simulink model "UAV_modelo_naolinear_1"  (R2017a)
settings: Solver=ode23s  StartTime=0.0  StopTime=T_sim  RelTol=1e-3  EnableMultiTasking=on
InitFcn:
  | main_modelo_nao_linear_v1
values from neighbouring files (symbols this model uses):
  dphi0 = 0    [main_model1.m]    (also in main_modelo_nao_linear_v1.m)
  dpsi0 = 0    [main_model1.m]    (also in main_modelo_nao_linear_v1.m)
  dtheta0 = 0    [main_model1.m]    (also in main_modelo_nao_linear_v1.m)
  g = 9.8    [main_model1.m]    (also in main_model2.m; main_modelo_linear_v1.m; main_modelo_linear_v2.m; main_modelo_nao_linear_v1.m)
  incluir_din_motor = -1    [main_model1.m]    (also in main_model2.m; main_modelo_nao_linear_v1.m = 1; main_modelo_nao_linear_v2.m; modelo_naolinear.m = 1)
  Ir = 1e-3    (= 0.001)    [main_model1.m]    (also in main_model2.m; main_modelo_linear_v1.m = 0.01; main_modelo_linear_v2.m = 0.01; main_modelo_nao_linear_v1.m)
  Ixx = 1e-2    (= 0.01)    [main_model1.m]    (also in main_model2.m; main_modelo_linear_v1.m; main_modelo_linear_v2.m; main_modelo_nao_linear_v1.m)
  Iyy = 1e-2    (= 0.01)    [main_model1.m]    (also in main_model2.m; main_modelo_linear_v1.m; main_modelo_linear_v2.m; main_modelo_nao_linear_v1.m)
  Izz = 1.8e-2    (= 0.018)    [main_model1.m]    (also in main_model2.m; main_modelo_linear_v1.m; main_modelo_linear_v2.m; main_modelo_nao_linear_v1.m)
  Kd_rot = 0.01    [main_model1.m]    (also in main_model2.m; main_modelo_linear_v1.m = 0; main_modelo_linear_v2.m = 0; main_modelo_nao_linear_v1.m)
  Kd_trans = 0.002    [main_model1.m]    (also in main_model2.m = -0.13723; main_modelo_linear_v1.m = 0; main_modelo_linear_v2.m = 0; main_modelo_nao_linear_v1.m)
  Ki_rot = 1.0    (= 1)    [main_model1.m]    (also in main_model2.m; main_modelo_linear_v1.m = 0.5; main_modelo_linear_v2.m = 0.5; main_modelo_nao_linear_v1.m)
  Ki_trans = 0.06    [main_model1.m]    (also in main_model2.m = 0.41774; main_modelo_linear_v1.m = 0; main_modelo_linear_v2.m = 1; main_modelo_nao_linear_v1.m)
  Kp = 0.9182    [main_model1.m]    (also in main_model2.m; main_modelo_nao_linear_v1.m; main_modelo_nao_linear_v2.m; modelo_naolinear.m)
  Kp_rot = 10    [main_model1.m]    (also in main_model2.m; main_modelo_linear_v1.m = 1; main_modelo_linear_v2.m = 1; main_modelo_nao_linear_v1.m)
  Kp_trans = 0.4    [main_model1.m]    (also in main_model2.m = 2.0968; main_modelo_linear_v1.m = 1; main_modelo_linear_v2.m = 2; main_modelo_nao_linear_v1.m)
  m = 1.0428    [main_model1.m]    (also in main_model2.m; main_modelo_linear_v1.m = 1; main_modelo_linear_v2.m = 1; main_modelo_nao_linear_v1.m)
  phi0 = 0    [main_model1.m]    (also in main_model2.m; main_modelo_linear_v1.m; main_modelo_linear_v2.m; main_modelo_nao_linear_v1.m)
  psi0 = 0    [main_model1.m]    (also in main_model2.m; main_modelo_linear_v1.m; main_modelo_linear_v2.m; main_modelo_nao_linear_v1.m)
  T = [kf,kf,kf,kf ... (first row only)    [main_model1.m]    (also in main_model2.m; main_modelo_nao_linear_v1.m; main_modelo_nao_linear_v2.m; modelo_naolinear.m)
  T_inv = T^(-1)    [main_model1.m]    (also in main_model2.m; main_modelo_nao_linear_v1.m; main_modelo_nao_linear_v2.m; modelo_naolinear.m)
  tau_a = 0.0569    [main_model1.m]    (also in main_model2.m; main_modelo_nao_linear_v1.m; main_modelo_nao_linear_v2.m; modelo_naolinear.m)
  tau_s = 0.0452    [main_model1.m]    (also in main_model2.m; main_modelo_nao_linear_v1.m; main_modelo_nao_linear_v2.m; modelo_naolinear.m)
  theta0 = 0    [main_model1.m]    (also in main_model2.m; main_modelo_linear_v1.m; main_modelo_linear_v2.m; main_modelo_nao_linear_v1.m)
  vx0 = 0    [main_model1.m]    (also in main_model2.m; main_modelo_nao_linear_v1.m; main_modelo_nao_linear_v2.m; modelo_naolinear.m)
  vxd = 0    [main_model1.m]    (also in main_model2.m; main_modelo_linear_v1.m; main_modelo_linear_v2.m; main_modelo_nao_linear_v1.m)
  vy0 = 0    [main_model1.m]    (also in main_model2.m; main_modelo_nao_linear_v1.m; main_modelo_nao_linear_v2.m; modelo_naolinear.m)
  vyd = 0    [main_model1.m]    (also in main_model2.m; main_modelo_linear_v1.m; main_modelo_linear_v2.m; main_modelo_nao_linear_v1.m)
  vz0 = 0    [main_model1.m]    (also in main_model2.m; main_modelo_nao_linear_v1.m; main_modelo_nao_linear_v2.m; modelo_naolinear.m)
  x0 = 0    [main_model1.m]    (also in main_model2.m; main_modelo_linear_v1.m; main_modelo_linear_v2.m; main_modelo_nao_linear_v1.m)
  y0 = 0    [main_model1.m]    (also in main_model2.m; main_modelo_linear_v1.m; main_modelo_linear_v2.m; main_modelo_nao_linear_v1.m)
  z0 = 1    [main_model1.m]    (also in main_model2.m; main_modelo_linear_v1.m; main_modelo_linear_v2.m; main_modelo_nao_linear_v1.m)
undefined symbols (not defined in the file or in its folder): sigbuilder_block
libraries: simulink x6, vrlib x2, aerolibutil x2, sharedutil x1
settings Model: Creator=dferr  LastModifiedBy=diego
settings DataIOCC: LimitDataPoints=on  SaveFormat=Array
settings OptimizationCC: LifeSpan=inf
settings DebuggingCC: SFUnexpectedBacktrackingDiag=warning  SFNoUnconditionalDefaultTransitionDiag=warning  SFExecutionAtInitializationDiag=none
settings HardwareCC: ProdBitPerPointer=32  ProdBitPerSizeT=32  ProdBitPerPtrDiffT=32  ProdLargestAtomicFloat=None  ProdIntDivRoundTo=Undefined  ProdEndianess=Unspecified  ProdWordSize=32  ProdHWDeviceType=32-bit Generic
settings ModelReferenceCC: PropagateSignalLabelsOutOfModel=off
settings GRTTargetCC: TargetLangStandard=C89/C90 (ANSI)  GeneratePreprocessorConditionals=Disable all
settings ConfigComp: CovMetricSettings=dw  CovHtmlReporting=on  CovSaveCumulativeToWorkspaceVar=on  CovSaveSingleToWorkspaceVar=on  CovExternalEMLEnable=off  CovSFcnEnable=off

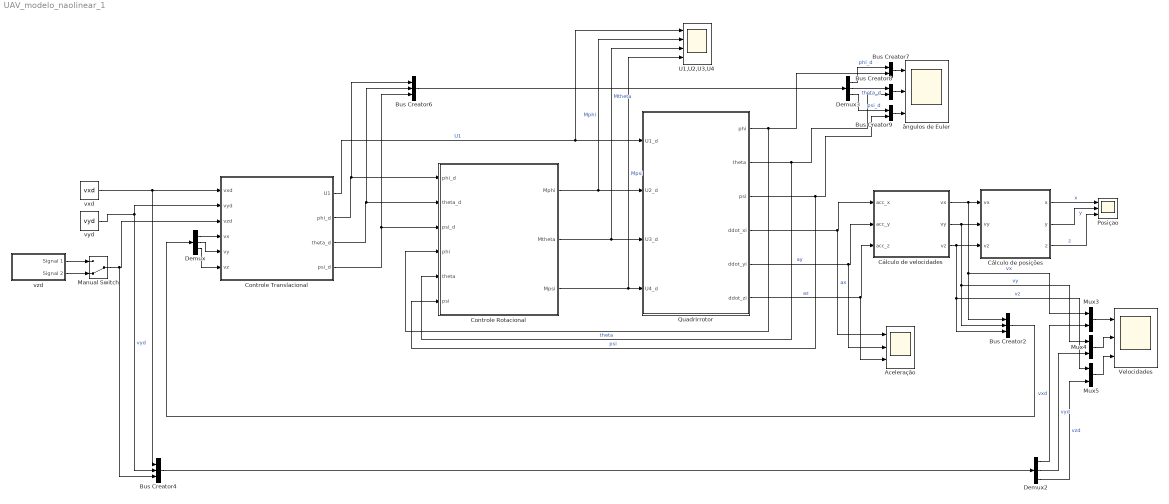
== system UAV_modelo_naolinear_1 ==
  Aceleração : Scope  NumInputPorts=3
  Bus Creator2 : BusCreator  Inputs=3
  Bus Creator4 : BusCreator  Inputs=3
  Bus Creator6 : BusCreator  Inputs=3
  Bus Creator7 : BusCreator  Inputs=2
  Bus Creator8 : BusCreator  Inputs=2
  Bus Creator9 : BusCreator  Inputs=2
  Controle Rotacional : Subsystem
      mask Display:
      | disp('Controle Rotacional')
      | port_label('input',1,'phi_d')
      | port_label('input',2,'theta_d')
      | port_label('input',3,'psi_d')
      | port_label('input',4,'phi')
      | port_label('input',5,'theta')
      | port_label('input',6,'psi')
      | port_label('output',1,'Mphi')
      | port_label('output',2,'Mtheta')
      | port_label('output',3,'Mpsi')
  Controle Translacional : Subsystem
      mask Display:
      | disp('Controle Translacional')
      | port_label('input',1,'vxd')
      | port_label('input',2,'vyd')
      | port_label('input',3,'vzd')
      | port_label('input',4,'vx')
      | port_label('input',5,'vy')
      | port_label('input',6,'vz')
      | port_label('output',1,'U1')
      | port_label('output',2,'phi_d')
      | port_label('output',3,'theta_d')
      | port_label('output',4,'psi_d')
  Cálculo de posições : Subsystem
      mask Display:
      | disp('Vel -> Pos')
      | port_label('input',1,'vel_x')
      | port_label('input',2,'vel_y')
      | port_label('input',3,'vel_ z')
      | port_label('output',1,'x')
      | port_label('output',2,'y')
      | port_label('output',3,'z')
  Cálculo de velocidades : Subsystem
      mask Display:
      | disp('Acc -> Vel')
      | port_label('input',1,'acc_x')
      | port_label('input',2,'acc_y')
      | port_label('input',3,'acc_z')
      | port_label('output',1,'vel_x')
      | port_label('output',2,'vel_y')
      | port_label('output',3,'vel_z')
  Demux : Demux  Outputs=3
  Demux2 : Demux  Outputs=3
  Demux3 : Demux  Outputs=3
  Manual Switch : ManualSwitch  CurrentSetting=0
  Mux3 : Mux  Inputs=2
  Mux4 : Mux  Inputs=2
  Mux5 : Mux  Inputs=2
  Posiçao : Scope  NumInputPorts=3
  Quadrirrotor : Subsystem
      mask Display:
      | disp('Quadrirrotor')
      | port_label('input',1,'U1')
      | port_label('input',2,'U2')
      | port_label('input',3,'U3')
      | port_label('input',4,'U4')
      | port_label('output',1,'phi')
      | port_label('output',2,'theta')
      | port_label('output',3,'psi')
      | port_label('output',4,'ddot_xi')
      | port_label('output',5,'ddot_yi')
      | port_label('output',6,'ddot_zi')
  U1,U2,U3,U4 : Scope  NumInputPorts=4
  Velocidades : Scope  NumInputPorts=3
  vxd : Constant  Value=vxd
  vyd : Constant  Value=vyd
  vzd : Subsystem  Tag=STV Subsys  LoadFcn=sigbuilder_block('load');  StartFcn=sigbuilder_block('start');  StopFcn=sigbuilder_block('stop');  ClipboardFcn=sigbuilder_block('clipboard');  mask(Sigbuilder block){tuvar=[0:10]}
      mask help: Simulink:masks:SigbuilderBlock_MD
      mask init:
      | if ~strcmp(get_param(bdroot(gcbh),'SimulationStatus'),'stopped') tuvar = sigbuilder_block('maskInit'); end
      settings: CopyFcn=sigbuilder_block('copy');  DeleteFcn=sigbuilder_block('delete');  ModelCloseFcn=sigbuilder_block('modelClose');  PreSaveFcn=sigbuilder_block('preSave');  PauseFcn=sigbuilder_block('pause');  ContinueFcn=sigbuilder_block('continue');  NameChangeFcn=sigbuilder_block('namechange');  OpenFcn=sigbuilder_block('open',[437.76 199.44 550.08 399.6 ]);  CloseFcn=sigbuilder_block('close');
      mask Display: plot(0, 0, 100, 100,[2, 2, 32, 32, 2], [68, 8, 8, 68, 68],[32, 2], [38, 38], [32, 19, 2],[53, 60, 44], [32, 17, 17, 2],[16, 16, 31, 31]);txt = getActiveGroup(gcbh);text(2, 100, txt,'verticalAlignment', 'top');
  ângulos de Euler : Scope  NumInputPorts=3
  wires:
  Cálculo de velocidades/1(vx) -> Mux3/1, Bus Creator2/1, Cálculo de posições/1(vx)  "vx"
  Cálculo de velocidades/2(vy) -> Mux4/1, Bus Creator2/2, Cálculo de posições/2(vy)  "vy"
  Cálculo de velocidades/3(vz) -> Mux5/1, Bus Creator2/3, Cálculo de posições/3(vz)  "vz"
  Bus Creator2/1 -> Demux/1
  vyd/1 -> Controle Translacional/2(vyd), Bus Creator4/2  "vyd"
  Mux3/1 -> Velocidades/1
  Mux4/1 -> Velocidades/2
  Mux5/1 -> Velocidades/3
  Bus Creator4/1 -> Demux2/1
  Demux2/1 -> Mux3/2  "vxd"
  Demux2/2 -> Mux4/2  "vyd"
  Demux2/3 -> Mux5/2  "vzd"
  Controle Rotacional/1(Mphi) -> U1,U2,U3,U4/2, Quadrirrotor/2(U2_d)  "Mphi"
  Controle Rotacional/2(Mtheta) -> U1,U2,U3,U4/3, Quadrirrotor/3(U3_d)  "Mtheta"
  Controle Rotacional/3(Mpsi) -> U1,U2,U3,U4/4, Quadrirrotor/4(U4_d)  "Mpsi"
  Quadrirrotor/1(phi) -> Controle Rotacional/4(phi), Bus Creator7/2
  Quadrirrotor/2(theta) -> Controle Rotacional/5(theta), Bus Creator8/2  "theta"
  Quadrirrotor/3(psi) -> Controle Rotacional/6(psi), Bus Creator9/2  "psi"
  Quadrirrotor/4(ddot_xi) -> Aceleração/1, Cálculo de velocidades/1(acc_x)  "ax"
  Quadrirrotor/5(ddot_yi) -> Aceleração/2, Cálculo de velocidades/2(acc_y)  "ay"
  Quadrirrotor/6(ddot_zi) -> Aceleração/3, Cálculo de velocidades/3(acc_z)  "az"
  Demux/1 -> Controle Translacional/4(vx)
  Demux/2 -> Controle Translacional/5(vy)
  Demux/3 -> Controle Translacional/6(vz)
  Controle Translacional/1(U1) -> U1,U2,U3,U4/1, Quadrirrotor/1(U1_d)  "U1"
  Controle Translacional/2(phi_d) -> Controle Rotacional/1(phi_d), Bus Creator6/1
  Controle Translacional/3(theta_d) -> Controle Rotacional/2(theta_d), Bus Creator6/2
  Controle Translacional/4(psi_d) -> Bus Creator6/3, Controle Rotacional/3(psi_d)
  Bus Creator6/1 -> Demux3/1
  Bus Creator7/1 -> ângulos de Euler/1
  Bus Creator8/1 -> ângulos de Euler/2
  Bus Creator9/1 -> ângulos de Euler/3
  Demux3/1 -> Bus Creator7/1  "phi_d"
  Demux3/2 -> Bus Creator8/1  "theta_d"
  Demux3/3 -> Bus Creator9/1  "psi_d"
  vxd/1 -> Bus Creator4/1, Controle Translacional/1(vxd)
  Cálculo de posições/1(x) -> Posiçao/1  "x"
  Cálculo de posições/2(y) -> Posiçao/2  "y"
  Cálculo de posições/3(z) -> Posiçao/3  "z"
  Manual Switch/1 -> Bus Creator4/3, Controle Translacional/3(vzd)
  vzd/1(Signal 1) -> Manual Switch/1
  vzd/2(Signal 2) -> Manual Switch/2

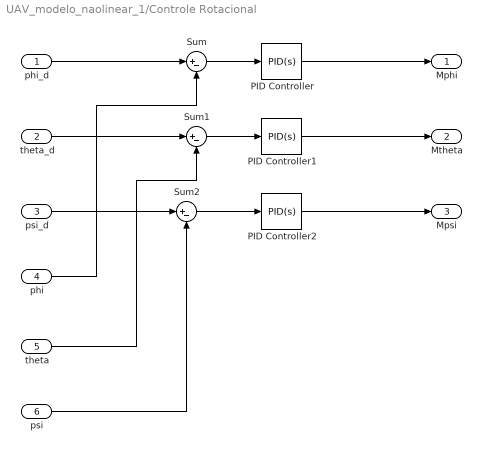
== system UAV_modelo_naolinear_1/Controle Rotacional ==
  phi_d : Inport
  theta_d : Inport  Port=2
  psi_d : Inport  Port=3
  phi : Inport  Port=4
  theta : Inport  Port=5
  psi : Inport  Port=6
  PID Controller : simulink/Continuous/PID Controller  Controller=PID  TimeDomain=Continuous-time  SampleTime=-1  IntegratorMethod=Forward Euler  FilterMethod=Forward Euler  Form=Parallel  UseFilter=on  ControllerParametersSource=internal  P=Kp_rot  I=Ki_rot  D=Kd_rot  N=100  InitialConditionSource=internal  InitialConditionForIntegrator=0  InitialConditionForFilter=0  ExternalReset=none  LimitOutput=off  UpperSaturationLimit=inf  LowerSaturationLimit=-inf  LinearizeAsGain=on  AntiWindupMode=none  Kb=1  TrackingMode=off  Kt=1  PParamMin=[]  PParamMax=[]  IParamMin=[]  IParamMax=[]  DParamMin=[]  DParamMax=[]  NParamMin=[]  NParamMax=[]  KbParamMin=[]  KbParamMax=[]  KtParamMin=[]  KtParamMax=[]  POutMin=[]  POutMax=[]  IOutMin=[]  IOutMax=[]  DOutMin=[]  DOutMax=[]  NOutMin=[]  NOutMax=[]  KbOutMin=[]  KbOutMax=[]  KtOutMin=[]  KtOutMax=[]  IntegratorOutMin=[]  IntegratorOutMax=[]  FilterOutMin=[]  FilterOutMax=[]  SumOutMin=[]  SumOutMax=[]  SumI1OutMin=[]  SumI1OutMax=[]  SumI2OutMin=[]  SumI2OutMax=[]  SumI3OutMin=[]  SumI3OutMax=[]  SumDOutMin=[]  SumDOutMax=[]  SaturationOutMin=[]  SaturationOutMax=[]  IntegratorContinuousStateAttributes=''  IntegratorStateMustResolveToSignalObject=off  IntegratorRTWStateStorageClass=Auto  FilterContinuousStateAttributes=''  FilterStateMustResolveToSignalObject=off  FilterRTWStateStorageClass=Auto  DifferentiatorICPrevScaledInput=0  DifferentiatorOutMin=[]  DifferentiatorOutMax=[]  InitialConditionSetting=State (most efficient)
  PID Controller1 : simulink/Continuous/PID Controller  Controller=PID  TimeDomain=Continuous-time  SampleTime=-1  IntegratorMethod=Forward Euler  FilterMethod=Forward Euler  Form=Parallel  UseFilter=on  ControllerParametersSource=internal  P=Kp_rot  I=Ki_rot  D=Kd_rot  N=100  InitialConditionSource=internal  InitialConditionForIntegrator=0  InitialConditionForFilter=0  ExternalReset=none  LimitOutput=off  UpperSaturationLimit=inf  LowerSaturationLimit=-inf  LinearizeAsGain=on  AntiWindupMode=none  Kb=1  TrackingMode=off  Kt=1  PParamMin=[]  PParamMax=[]  IParamMin=[]  IParamMax=[]  DParamMin=[]  DParamMax=[]  NParamMin=[]  NParamMax=[]  KbParamMin=[]  KbParamMax=[]  KtParamMin=[]  KtParamMax=[]  POutMin=[]  POutMax=[]  IOutMin=[]  IOutMax=[]  DOutMin=[]  DOutMax=[]  NOutMin=[]  NOutMax=[]  KbOutMin=[]  KbOutMax=[]  KtOutMin=[]  KtOutMax=[]  IntegratorOutMin=[]  IntegratorOutMax=[]  FilterOutMin=[]  FilterOutMax=[]  SumOutMin=[]  SumOutMax=[]  SumI1OutMin=[]  SumI1OutMax=[]  SumI2OutMin=[]  SumI2OutMax=[]  SumI3OutMin=[]  SumI3OutMax=[]  SumDOutMin=[]  SumDOutMax=[]  SaturationOutMin=[]  SaturationOutMax=[]  IntegratorContinuousStateAttributes=''  IntegratorStateMustResolveToSignalObject=off  IntegratorRTWStateStorageClass=Auto  FilterContinuousStateAttributes=''  FilterStateMustResolveToSignalObject=off  FilterRTWStateStorageClass=Auto  DifferentiatorICPrevScaledInput=0  DifferentiatorOutMin=[]  DifferentiatorOutMax=[]  InitialConditionSetting=State (most efficient)
  PID Controller2 : simulink/Continuous/PID Controller  Controller=PID  TimeDomain=Continuous-time  SampleTime=-1  IntegratorMethod=Forward Euler  FilterMethod=Forward Euler  Form=Parallel  UseFilter=on  ControllerParametersSource=internal  P=Kp_rot  I=Ki_rot  D=Kd_rot  N=100  InitialConditionSource=internal  InitialConditionForIntegrator=0  InitialConditionForFilter=0  ExternalReset=none  LimitOutput=off  UpperSaturationLimit=inf  LowerSaturationLimit=-inf  LinearizeAsGain=on  AntiWindupMode=none  Kb=1  TrackingMode=off  Kt=1  PParamMin=[]  PParamMax=[]  IParamMin=[]  IParamMax=[]  DParamMin=[]  DParamMax=[]  NParamMin=[]  NParamMax=[]  KbParamMin=[]  KbParamMax=[]  KtParamMin=[]  KtParamMax=[]  POutMin=[]  POutMax=[]  IOutMin=[]  IOutMax=[]  DOutMin=[]  DOutMax=[]  NOutMin=[]  NOutMax=[]  KbOutMin=[]  KbOutMax=[]  KtOutMin=[]  KtOutMax=[]  IntegratorOutMin=[]  IntegratorOutMax=[]  FilterOutMin=[]  FilterOutMax=[]  SumOutMin=[]  SumOutMax=[]  SumI1OutMin=[]  SumI1OutMax=[]  SumI2OutMin=[]  SumI2OutMax=[]  SumI3OutMin=[]  SumI3OutMax=[]  SumDOutMin=[]  SumDOutMax=[]  SaturationOutMin=[]  SaturationOutMax=[]  IntegratorContinuousStateAttributes=''  IntegratorStateMustResolveToSignalObject=off  IntegratorRTWStateStorageClass=Auto  FilterContinuousStateAttributes=''  FilterStateMustResolveToSignalObject=off  FilterRTWStateStorageClass=Auto  DifferentiatorICPrevScaledInput=0  DifferentiatorOutMin=[]  DifferentiatorOutMax=[]  InitialConditionSetting=State (most efficient)
  Sum : Sum  Inputs=|+-
  Sum1 : Sum  Inputs=|+-
  Sum2 : Sum  Inputs=|+-
  Mphi : Outport
  Mtheta : Outport  Port=2
  Mpsi : Outport  Port=3
  wires:
  Sum/1 -> PID Controller/1
  phi_d/1 -> Sum/1
  Sum1/1 -> PID Controller1/1
  Sum2/1 -> PID Controller2/1
  theta_d/1 -> Sum1/1
  psi_d/1 -> Sum2/1
  phi/1 -> Sum/2
  theta/1 -> Sum1/2
  psi/1 -> Sum2/2
  PID Controller/1 -> Mphi/1
  PID Controller1/1 -> Mtheta/1
  PID Controller2/1 -> Mpsi/1

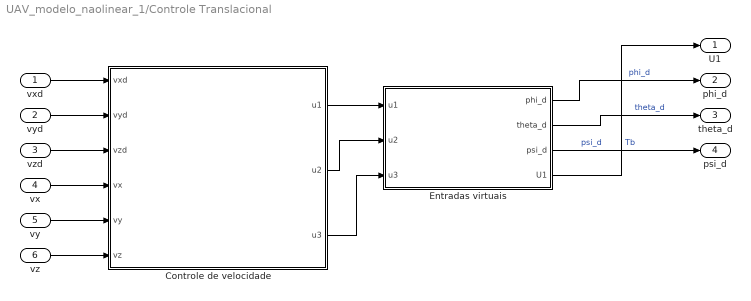
== system UAV_modelo_naolinear_1/Controle Translacional ==
  vxd : Inport
  vyd : Inport  Port=2
  vzd : Inport  Port=3
  vx : Inport  Port=4
  vy : Inport  Port=5
  vz : Inport  Port=6
  Controle de velocidade : Subsystem
      mask Display:
      | disp('Controle de Velocidade PID')
      | port_label('input',1,'vxd')
      | port_label('input',2,'vyd')
      | port_label('input',3,'vzd')
      | port_label('input',4,'vx')
      | port_label('input',5,'vy')
      | port_label('input',6,'vz')
      | 
      | port_label('output',1,'u1')
      | port_label('output',2,'u2')
      | port_label('output',3,'u3')
  Entradas virtuais : Subsystem
      mask Display:
      | disp('(u1,u2,u3)->(eta_d,U1)')
      | port_label('input',1,'u1')
      | port_label('input',2,'u2')
      | port_label('input',3,'u3')
      | port_label('output',1,'phi_d')
      | port_label('output',2,'theta_d')
      | port_label('output',3,'psi_d')
      | port_label('output',4,'U1')
  U1 : Outport
  phi_d : Outport  Port=2
  theta_d : Outport  Port=3
  psi_d : Outport  Port=4
  wires:
  Controle de velocidade/2(u2) -> Entradas virtuais/2(u2)
  Entradas virtuais/1(phi_d) -> phi_d/1  "phi_d"
  Entradas virtuais/2(theta_d) -> theta_d/1  "theta_d"
  Entradas virtuais/3(psi_d) -> psi_d/1  "psi_d"
  Controle de velocidade/1(u1) -> Entradas virtuais/1(u1)
  vz/1 -> Controle de velocidade/6(vz)
  vy/1 -> Controle de velocidade/5("vy ")
  Controle de velocidade/3(u3) -> Entradas virtuais/3(u3)
  vx/1 -> Controle de velocidade/4(vx)
  Entradas virtuais/4(U1) -> U1/1  "Tb"
  vyd/1 -> Controle de velocidade/2(vyd)
  vzd/1 -> Controle de velocidade/3(vzd)
  vxd/1 -> Controle de velocidade/1(vxd)

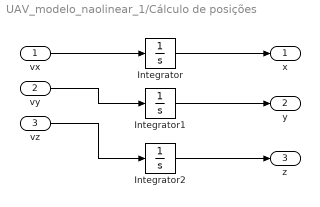
== system UAV_modelo_naolinear_1/Cálculo de posições ==
  vx : Inport
  vy : Inport  Port=2
  vz : Inport  Port=3
  Integrator : Integrator  InitialCondition=x0
  Integrator1 : Integrator  InitialCondition=y0
  Integrator2 : Integrator  InitialCondition=z0  LimitOutput=on  LowerSaturationLimit=0
  x : Outport
  y : Outport  Port=2
  z : Outport  Port=3
  wires:
  Integrator/1 -> x/1
  Integrator1/1 -> y/1
  vy/1 -> Integrator1/1
  vz/1 -> Integrator2/1
  vx/1 -> Integrator/1
  Integrator2/1 -> z/1

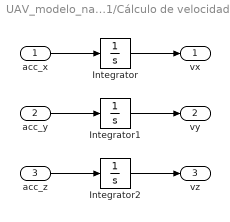
== system UAV_modelo_naolinear_1/Cálculo de velocidades ==
  acc_x : Inport
  acc_y : Inport  Port=2
  acc_z : Inport  Port=3
  Integrator : Integrator  InitialCondition=vx0  ZeroCross=off
  Integrator1 : Integrator  InitialCondition=vy0  ZeroCross=off
  Integrator2 : Integrator  InitialCondition=vz0  ZeroCross=off
  vx : Outport
  vy : Outport  Port=2
  vz : Outport  Port=3
  wires:
  Integrator2/1 -> vz/1
  acc_z/1 -> Integrator2/1
  Integrator/1 -> vx/1
  acc_x/1 -> Integrator/1
  acc_y/1 -> Integrator1/1
  Integrator1/1 -> vy/1

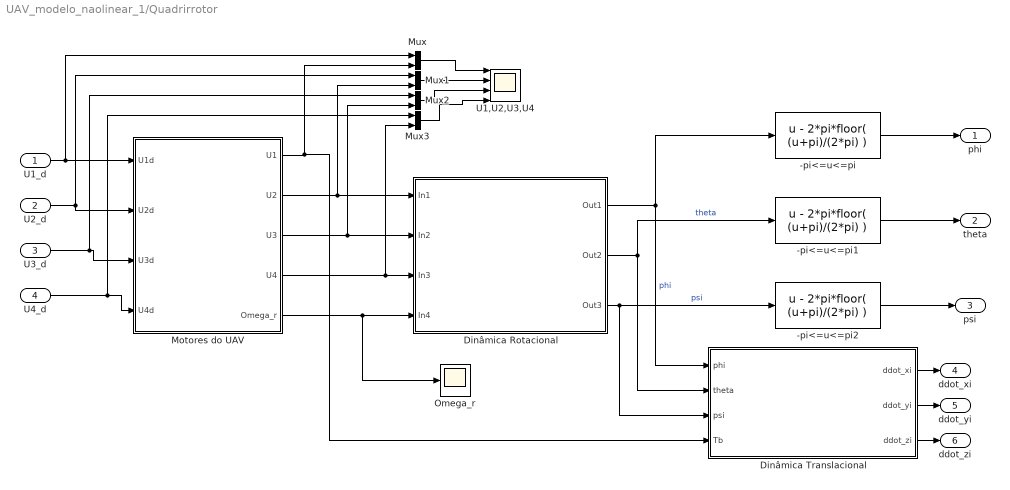
== system UAV_modelo_naolinear_1/Quadrirrotor ==
  U1_d : Inport
  U2_d : Inport  Port=2
  U3_d : Inport  Port=3
  U4_d : Inport  Port=4
  -pi<=u<=pi : Fcn  Expr=u - 2*pi*floor( (u+pi)/(2*pi) )
  -pi<=u<=pi1 : Fcn  Expr=u - 2*pi*floor( (u+pi)/(2*pi) )
  -pi<=u<=pi2 : Fcn  Expr=u - 2*pi*floor( (u+pi)/(2*pi) )
  Dinâmica Rotacional : Subsystem
      mask Display:
      | disp('Dinâmica Rotacional')
      | port_label('input',1,'Mphi')
      | port_label('input',2,'Mtheta')
      | port_label('input',3,'Mpsi')
      | port_label('input',4,'Omega_r')
      | port_label('output',1,'phi')
      | port_label('output',2,'theta')
      | port_label('output',3,'psi')
  Dinâmica Translacional : Subsystem
      mask Display:
      | disp ('Dinâmica Translacional')
      | port_label('input',1,'phi')
      | port_label('input',2,'theta')
      | port_label('input',3,'psi')
      | port_label('input',4,'Tb')
      | port_label('output',1,'ddot_xi')
      | port_label('output',2,'ddot_yi')
      | port_label('output',3,'ddot_zi')
  "Motores do UAV " : Subsystem
      mask Display:
      | disp('Dinâmica Motores')
      | port_label('input',1,'U1d')
      | port_label('input',2,'U2d')
      | port_label('input',3,'U3d')
      | port_label('input',4,'U4d')
      | port_label('output',1,'U1')
      | port_label('output',2,'U2')
      | port_label('output',3,'U3')
      | port_label('output',4,'U4')
      | port_label('output',5,'Omega_r')
  Mux{,1..3} (4 alike) : Mux  Inputs=2
  Omega_r : Scope
  U1,U2,U3,U4 : Scope  NumInputPorts=4
  phi : Outport
  theta : Outport  Port=2
  psi : Outport  Port=3
  ddot_xi : Outport  Port=4
  ddot_yi : Outport  Port=5
  ddot_zi : Outport  Port=6
  wires:
  Dinâmica Rotacional/3(Out3) -> Dinâmica Translacional/3(psi), -pi<=u<=pi2/1  "psi"
  Dinâmica Rotacional/2(Out2) -> Dinâmica Translacional/2(theta), -pi<=u<=pi1/1  "theta"
  Dinâmica Rotacional/1(Out1) -> Dinâmica Translacional/1(phi), -pi<=u<=pi/1  "phi"
  Dinâmica Translacional/1(ddot_xi) -> ddot_xi/1
  Dinâmica Translacional/2(ddot_yi) -> ddot_yi/1
  Dinâmica Translacional/3(ddot_zi) -> ddot_zi/1
  U2_d/1 -> "Motores do UAV "/2(U2d), Mux1/1
  U3_d/1 -> "Motores do UAV "/3(U3d), Mux2/1
  Mux/1 -> U1,U2,U3,U4/1
  Mux1/1 -> U1,U2,U3,U4/2
  Mux2/1 -> U1,U2,U3,U4/3
  Mux3/1 -> U1,U2,U3,U4/4
  "Motores do UAV "/3(U3) -> Dinâmica Rotacional/2(In2), Mux2/2
  "Motores do UAV "/4(U4) -> Mux3/2, Dinâmica Rotacional/3(In3)
  "Motores do UAV "/2(U2) -> Dinâmica Rotacional/1(In1), Mux1/2
  "Motores do UAV "/1(U1) -> Mux/2, Dinâmica Translacional/4(Tb)
  U1_d/1 -> "Motores do UAV "/1(U1d), Mux/1
  U4_d/1 -> "Motores do UAV "/4(U4d), Mux3/1
  "Motores do UAV "/5(Omega_r) -> Omega_r/1, Dinâmica Rotacional/4(In4)
  -pi<=u<=pi/1 -> phi/1
  -pi<=u<=pi1/1 -> theta/1
  -pi<=u<=pi2/1 -> psi/1

== system UAV_modelo_naolinear_1/vzd ==
  Demux : Demux  Tag=STV Demux  Outputs=2
  FromWs : FromWorkspace  Tag=STV FromWs  VariableName=tuvar  SampleTime=0
      SigBuilderData=|
      | common.afterFinalStr = 'Extrapolate'
      | common.sampleTime = 0
      | dataSet.timeRange = [0 20]
      | dataSet.name = 'Group 1'
      | sbobj.Groups.Name = 'Group 1'
      | sbobj.Groups.Signals(1).Name = 'Signal 1'
      | sbobj.Groups.Signals(1).XData = [0 2.05 4.75 8 18 20]
      | sbobj.Groups.Signals(1).YData = [-0.2 8.5 20 20 0 0]
      | sbobj.Groups.Signals(2).Name = 'Signal 2'
      | sbobj.Groups.Signals(2).XData = [0 5 5 20]
      | sbobj.Groups.Signals(2).YData = [0 0 1 1]
      | sbobj.Groups.TimeRange = [0 20]
  Signal 1 : Outport  Tag=STV Outport
  Signal 2 : Outport  Tag=STV Outport  Port=2
  wires:
  FromWs/1 -> Demux/1
  Demux/1 -> Signal 1/1
  Demux/2 -> Signal 2/1

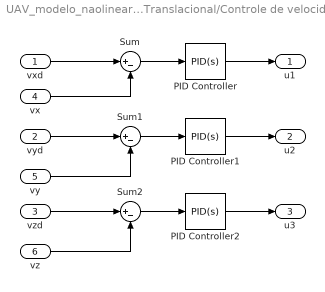
== system UAV_modelo_naolinear_1/Controle Translacional/Controle de velocidade ==
  vxd : Inport
  vyd : Inport  Port=2
  vzd : Inport  Port=3
  vx : Inport  Port=4
  "vy " : Inport  Port=5
  vz : Inport  Port=6
  PID Controller : simulink/Continuous/PID Controller  Controller=PID  TimeDomain=Continuous-time  SampleTime=-1  IntegratorMethod=Forward Euler  FilterMethod=Forward Euler  Form=Parallel  UseFilter=on  ControllerParametersSource=internal  P=Kp_trans  I=Ki_trans  D=Kd_trans  N=100  InitialConditionSource=internal  InitialConditionForIntegrator=0  InitialConditionForFilter=0  ExternalReset=none  LimitOutput=off  UpperSaturationLimit=inf  LowerSaturationLimit=-inf  LinearizeAsGain=on  AntiWindupMode=none  Kb=1  TrackingMode=off  Kt=1  RndMeth=Nearest  PParamMin=[]  PParamMax=[]  IParamMin=[]  IParamMax=[]  DParamMin=[]  DParamMax=[]  NParamMin=[]  NParamMax=[]  KbParamMin=[]  KbParamMax=[]  KtParamMin=[]  KtParamMax=[]  POutMin=[]  POutMax=[]  IOutMin=[]  IOutMax=[]  DOutMin=[]  DOutMax=[]  NOutMin=[]  NOutMax=[]  KbOutMin=[]  KbOutMax=[]  KtOutMin=[]  KtOutMax=[]  IntegratorOutMin=[]  IntegratorOutMax=[]  FilterOutMin=[]  FilterOutMax=[]  SumOutMin=[]  SumOutMax=[]  SumI1OutMin=[]  SumI1OutMax=[]  SumI2OutMin=[]  SumI2OutMax=[]  SumI3OutMin=[]  SumI3OutMax=[]  SumDOutMin=[]  SumDOutMax=[]  SaturationOutMin=[]  SaturationOutMax=[]  IntegratorContinuousStateAttributes=''  IntegratorStateMustResolveToSignalObject=off  IntegratorRTWStateStorageClass=Auto  FilterContinuousStateAttributes=''  FilterStateMustResolveToSignalObject=off  FilterRTWStateStorageClass=Auto  DifferentiatorICPrevScaledInput=0  DifferentiatorOutMin=[]  DifferentiatorOutMax=[]  InitialConditionSetting=State (most efficient)
      settings: LockScale=on
  PID Controller1 : simulink/Continuous/PID Controller  Controller=PID  TimeDomain=Continuous-time  SampleTime=-1  IntegratorMethod=Forward Euler  FilterMethod=Forward Euler  Form=Parallel  UseFilter=on  ControllerParametersSource=internal  P=Kp_trans  I=Ki_trans  D=Kd_trans  N=100  InitialConditionSource=internal  InitialConditionForIntegrator=0  InitialConditionForFilter=0  ExternalReset=none  LimitOutput=off  UpperSaturationLimit=inf  LowerSaturationLimit=-inf  LinearizeAsGain=on  AntiWindupMode=none  Kb=1  TrackingMode=off  Kt=1  RndMeth=Nearest  PParamMin=[]  PParamMax=[]  IParamMin=[]  IParamMax=[]  DParamMin=[]  DParamMax=[]  NParamMin=[]  NParamMax=[]  KbParamMin=[]  KbParamMax=[]  KtParamMin=[]  KtParamMax=[]  POutMin=[]  POutMax=[]  IOutMin=[]  IOutMax=[]  DOutMin=[]  DOutMax=[]  NOutMin=[]  NOutMax=[]  KbOutMin=[]  KbOutMax=[]  KtOutMin=[]  KtOutMax=[]  IntegratorOutMin=[]  IntegratorOutMax=[]  FilterOutMin=[]  FilterOutMax=[]  SumOutMin=[]  SumOutMax=[]  SumI1OutMin=[]  SumI1OutMax=[]  SumI2OutMin=[]  SumI2OutMax=[]  SumI3OutMin=[]  SumI3OutMax=[]  SumDOutMin=[]  SumDOutMax=[]  SaturationOutMin=[]  SaturationOutMax=[]  IntegratorContinuousStateAttributes=''  IntegratorStateMustResolveToSignalObject=off  IntegratorRTWStateStorageClass=Auto  FilterContinuousStateAttributes=''  FilterStateMustResolveToSignalObject=off  FilterRTWStateStorageClass=Auto  DifferentiatorICPrevScaledInput=0  DifferentiatorOutMin=[]  DifferentiatorOutMax=[]  InitialConditionSetting=State (most efficient)
      settings: LockScale=on
  PID Controller2 : simulink/Continuous/PID Controller  Controller=PID  TimeDomain=Continuous-time  SampleTime=-1  IntegratorMethod=Forward Euler  FilterMethod=Forward Euler  Form=Parallel  UseFilter=on  ControllerParametersSource=internal  P=Kp_trans  I=Ki_trans  D=Kd_trans  N=100  InitialConditionSource=internal  InitialConditionForIntegrator=0  InitialConditionForFilter=0  ExternalReset=none  LimitOutput=off  UpperSaturationLimit=inf  LowerSaturationLimit=-inf  LinearizeAsGain=on  AntiWindupMode=none  Kb=1  TrackingMode=off  Kt=1  RndMeth=Nearest  PParamMin=[]  PParamMax=[]  IParamMin=[]  IParamMax=[]  DParamMin=[]  DParamMax=[]  NParamMin=[]  NParamMax=[]  KbParamMin=[]  KbParamMax=[]  KtParamMin=[]  KtParamMax=[]  POutMin=[]  POutMax=[]  IOutMin=[]  IOutMax=[]  DOutMin=[]  DOutMax=[]  NOutMin=[]  NOutMax=[]  KbOutMin=[]  KbOutMax=[]  KtOutMin=[]  KtOutMax=[]  IntegratorOutMin=[]  IntegratorOutMax=[]  FilterOutMin=[]  FilterOutMax=[]  SumOutMin=[]  SumOutMax=[]  SumI1OutMin=[]  SumI1OutMax=[]  SumI2OutMin=[]  SumI2OutMax=[]  SumI3OutMin=[]  SumI3OutMax=[]  SumDOutMin=[]  SumDOutMax=[]  SaturationOutMin=[]  SaturationOutMax=[]  IntegratorContinuousStateAttributes=''  IntegratorStateMustResolveToSignalObject=off  IntegratorRTWStateStorageClass=Auto  FilterContinuousStateAttributes=''  FilterStateMustResolveToSignalObject=off  FilterRTWStateStorageClass=Auto  DifferentiatorICPrevScaledInput=0  DifferentiatorOutMin=[]  DifferentiatorOutMax=[]  InitialConditionSetting=State (most efficient)
      settings: LockScale=on
  Sum : Sum  Inputs=|+-
  Sum1 : Sum  Inputs=|+-
  Sum2 : Sum  Inputs=|+-
  u1 : Outport
  u2 : Outport  Port=2
  u3 : Outport  Port=3
  wires:
  vxd/1 -> Sum/1
  vz/1 -> Sum2/2
  vyd/1 -> Sum1/1
  vzd/1 -> Sum2/1
  vx/1 -> Sum/2
  "vy "/1 -> Sum1/2
  Sum/1 -> PID Controller/1
  PID Controller/1 -> u1/1
  Sum2/1 -> PID Controller2/1
  PID Controller2/1 -> u3/1
  PID Controller1/1 -> u2/1
  Sum1/1 -> PID Controller1/1

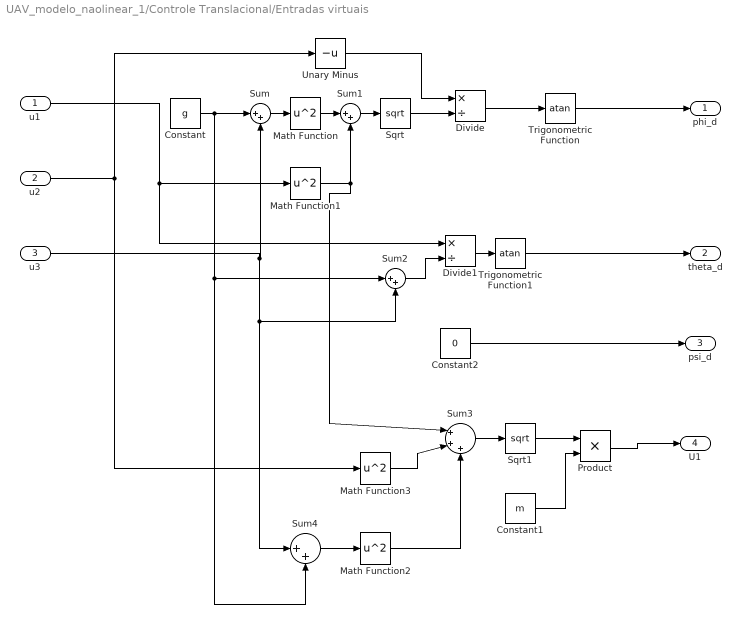
== system UAV_modelo_naolinear_1/Controle Translacional/Entradas virtuais ==
  u1 : Inport
  u2 : Inport  Port=2
  u3 : Inport  Port=3
  Constant : Constant  Value=g
  Constant1 : Constant  Value=m
  Constant2 : Constant  Value=0
  Divide : Product  Inputs=*/
  Divide1 : Product  Inputs=*/
  Math Function{,1..3} (4 alike) : Math  Operator=square  SaturateOnIntegerOverflow=on
  Product : Product
  Sqrt : Sqrt  SaturateOnIntegerOverflow=on
  Sqrt1 : Sqrt  SaturateOnIntegerOverflow=on
  Sum{,1..2,4} (4 alike) : Sum  Inputs=|++
  Sum3 : Sum  Inputs=|+++
  Trigonometric Function : Trigonometry  Operator=atan
  Trigonometric Function1 : Trigonometry  Operator=atan
  Unary Minus : UnaryMinus
  phi_d : Outport
  theta_d : Outport  Port=2
  psi_d : Outport  Port=3
  U1 : Outport  Port=4
  wires:
  Divide/1 -> Trigonometric Function/1
  Sqrt/1 -> Divide/2
  Trigonometric Function1/1 -> theta_d/1
  Sum1/1 -> Sqrt/1
  Divide1/1 -> Trigonometric Function1/1
  Sum/1 -> Math Function/1
  u1/1 -> Divide1/1, Math Function1/1
  Trigonometric Function/1 -> phi_d/1
  Sum2/1 -> Divide1/2
  Constant1/1 -> Product/2
  Math Function3/1 -> Sum3/2
  u2/1 -> Math Function3/1, Unary Minus/1
  Constant2/1 -> psi_d/1
  Sqrt1/1 -> Product/1
  Sum3/1 -> Sqrt1/1
  Math Function2/1 -> Sum3/3
  u3/1 -> Sum4/1, Sum2/2, Sum/2
  Constant/1 -> Sum4/2, Sum2/1, Sum/1
  Math Function/1 -> Sum1/1
  Product/1 -> U1/1
  Math Function1/1 -> Sum3/1, Sum1/2
  Sum4/1 -> Math Function2/1
  Unary Minus/1 -> Divide/1

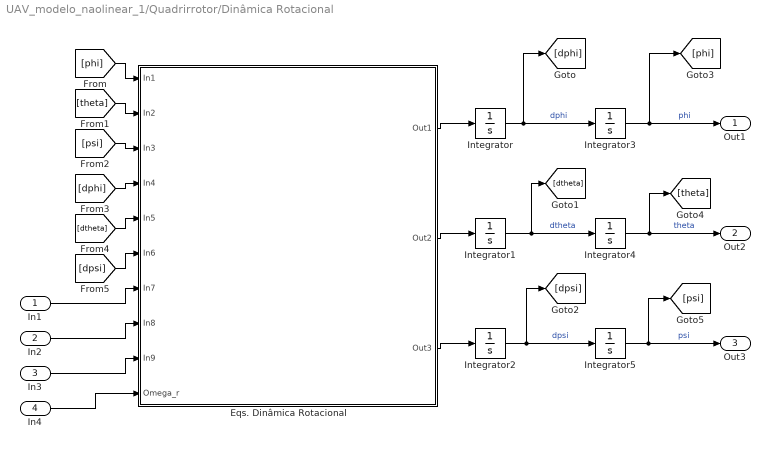
== system UAV_modelo_naolinear_1/Quadrirrotor/Dinâmica Rotacional ==
  In1 : Inport
  In2 : Inport  Port=2
  In3 : Inport  Port=3
  In4 : Inport  Port=4
  Eqs. Dinâmica Rotacional : Subsystem
      mask Display:
      | disp('Eqs. Dinâmica Rotacional')
      | port_label('input',1,'phi')
      | port_label('input',2,'theta')
      | port_label('input',3,'psi')
      | port_label('input',4,'dphi')
      | port_label('input',5,'dtheta')
      | port_label('input',6,'dpsi')
      | port_label('input',7,'Mphi')
      | port_label('input',8,'Mtheta')
      | port_label('input',9,'Mpsi')
      | port_label('input',10,'Omega_r')
      | port_label('output',1,'ddphi')
      | port_label('output',2,'ddtheta')
      | port_label('output',3,'ddpsi')
  Integrator : Integrator  InitialCondition=dphi0
  Integrator1 : Integrator  InitialCondition=dtheta0
  Integrator2 : Integrator  InitialCondition=dpsi0
  Integrator3 : Integrator  InitialCondition=phi0
  Integrator4 : Integrator  InitialCondition=theta0
  Integrator5 : Integrator  InitialCondition=psi0
  Out1 : Outport
  Out2 : Outport  Port=2
  Out3 : Outport  Port=3
  wires:
  Integrator5/1 -> [psi], Out3/1  "psi"
  Eqs. Dinâmica Rotacional/3(Out3) -> Integrator2/1
  In1/1 -> Eqs. Dinâmica Rotacional/7(In7)
  Integrator3/1 -> [phi], Out1/1  "phi"
  Integrator1/1 -> [dtheta], Integrator4/1  "dtheta"
  Integrator2/1 -> [dpsi], Integrator5/1  "dpsi"
  In3/1 -> Eqs. Dinâmica Rotacional/9(In9)
  Integrator4/1 -> [theta], Out2/1  "theta"
  In2/1 -> Eqs. Dinâmica Rotacional/8(In8)
  Integrator/1 -> [dphi], Integrator3/1  "dphi"
  Eqs. Dinâmica Rotacional/1(Out1) -> Integrator/1
  Eqs. Dinâmica Rotacional/2(Out2) -> Integrator1/1
  [phi] -> Eqs. Dinâmica Rotacional/1(In1)
  [theta] -> Eqs. Dinâmica Rotacional/2(In2)
  [psi] -> Eqs. Dinâmica Rotacional/3(In3)
  [dphi] -> Eqs. Dinâmica Rotacional/4(In4)
  [dtheta] -> Eqs. Dinâmica Rotacional/5(In5)
  [dpsi] -> Eqs. Dinâmica Rotacional/6(In6)
  In4/1 -> Eqs. Dinâmica Rotacional/10(Omega_r)

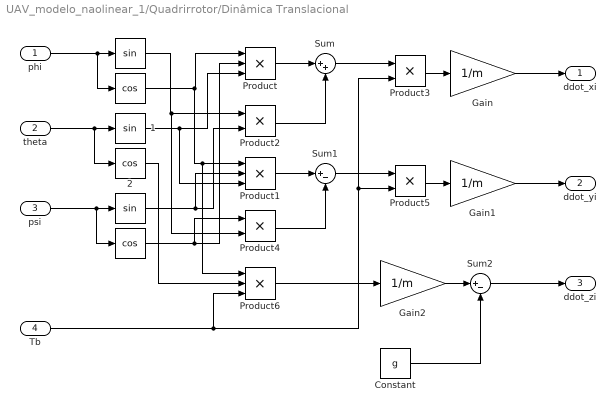
== system UAV_modelo_naolinear_1/Quadrirrotor/Dinâmica Translacional ==
  phi : Inport
  theta : Inport  Port=2
  psi : Inport  Port=3
  Tb : Inport  Port=4
  " " : Trigonometry
  "  " : Trigonometry  Operator=cos
  "   " : Trigonometry  Operator=cos
  "    " : Trigonometry  Operator=cos
  " 1" : Trigonometry
  " 2" : Trigonometry
  Constant : Constant  Value=g
  Gain : Gain  Gain=1/m
  Gain1 : Gain  Gain=1/m
  Gain2 : Gain  Gain=1/m
  Product : Product  Inputs=3
  Product1 : Product  Inputs=3
  Product{2..5} (4 alike) : Product
  Product6 : Product  Inputs=3
  Sum : Sum  Inputs=|++
  Sum1 : Sum  Inputs=|+-
  Sum2 : Sum  Inputs=|+-
  ddot_xi : Outport
  ddot_yi : Outport  Port=2
  ddot_zi : Outport  Port=3
  wires:
  Product6/1 -> Gain2/1
  Product3/1 -> Gain/1
  Sum2/1 -> ddot_zi/1
  " 1"/1 -> Product1/3, Product/3
  Product1/1 -> Sum1/1
  phi/1 -> "  "/1, " "/1
  " 2"/1 -> Product1/2, Product2/2
  "    "/1 -> Product4/1, Product/2
  Sum/1 -> Product3/1
  Product2/1 -> Sum/2
  " "/1 -> Product4/2, Product2/1
  Constant/1 -> Sum2/2
  Gain1/1 -> ddot_yi/1
  theta/1 -> "   "/1, " 1"/1
  Product5/1 -> Gain1/1
  psi/1 -> "    "/1, " 2"/1
  Tb/1 -> Product5/2, Product3/2, Product6/3
  Product/1 -> Sum/1
  Product4/1 -> Sum1/2
  Gain2/1 -> Sum2/1
  "   "/1 -> Product6/2
  "  "/1 -> Product6/1, Product1/1, Product/1
  Gain/1 -> ddot_xi/1
  Sum1/1 -> Product5/1

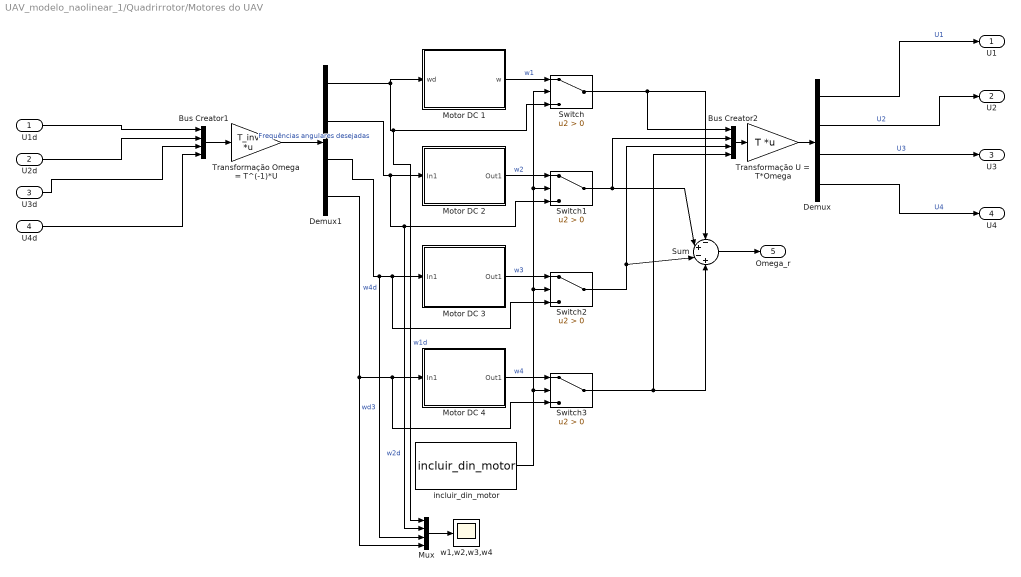
== system UAV_modelo_naolinear_1/Quadrirrotor/Motores do UAV  ==
  U1d : Inport
  U2d : Inport  Port=2
  U3d : Inport  Port=3
  U4d : Inport  Port=4
  Bus Creator1 : BusCreator  Inputs=4
  Bus Creator2 : BusCreator  Inputs=4
  Demux : Demux
  Demux1 : Demux
  Motor DC 1 : Subsystem
      mask Display:
      | disp('Motor DC')
      | port_label('input',1,'wd')
      | port_label('output',1,'w')
  Motor DC 2 : Subsystem
      mask Display:
      | disp('Motod DC')
      | port_label('input',1,'wd')
      | port_label('output',1,'w')
  Motor DC 3 : Subsystem
      mask Display:
      | disp('Motod DC')
      | port_label('input',1,'wd')
      | port_label('output',1,'w')
  Motor DC 4 : Subsystem
      mask Display:
      | disp('Motod DC')
      | port_label('input',1,'wd')
      | port_label('output',1,'w')
  Mux : Mux
  Sum : Sum  Inputs=-+-+
  Switch{,1..3} (4 alike) : Switch  Criteria=u2 > Threshold
  Transformação Omega = T^(-1)*U : Gain  Gain=T_inv  Multiplication=Matrix(K*u)  RndMeth=Nearest  LockScale=on
  Transformação U = T*Omega : Gain  Gain=T  Multiplication=Matrix(K*u)  RndMeth=Nearest  LockScale=on
  incluir_din_motor : Constant  Value=incluir_din_motor
  w1,w2,w3,w4 : Scope
  U1 : Outport
  U2 : Outport  Port=2
  U3 : Outport  Port=3
  U4 : Outport  Port=4
  Omega_r : Outport  Port=5
  wires:
  Demux1/1 -> Motor DC 1/1(wd), Mux/1, Switch/3  "w1d"
  Bus Creator2/1 -> Transformação U = T*Omega/1
  Transformação Omega = T^(-1)*U/1 -> Demux1/1  "Frequências angulares desejadas"
  Transformação U = T*Omega/1 -> Demux/1
  Demux/4 -> U4/1  "U4"
  Demux/3 -> U3/1  "U3"
  Bus Creator1/1 -> Transformação Omega = T^(-1)*U/1
  Demux/2 -> U2/1  "U2"
  Demux/1 -> U1/1  "U1"
  Sum/1 -> Omega_r/1
  Demux1/2 -> Mux/2, Switch1/3, Motor DC 2/1(In1)  "w2d"
  Demux1/3 -> Mux/3, Switch2/3, Motor DC 3/1(In1)  "wd3"
  Demux1/4 -> Mux/4, Switch3/3, Motor DC 4/1(In1)  "w4d"
  Switch/1 -> Sum/1, Bus Creator2/1
  Motor DC 1/1(w) -> Switch/1  "w1"
  Motor DC 2/1(Out1) -> Switch1/1  "w2"
  Switch1/1 -> Sum/2, Bus Creator2/2
  Motor DC 3/1(Out1) -> Switch2/1  "w3"
  Switch2/1 -> Sum/3, Bus Creator2/3
  Motor DC 4/1(Out1) -> Switch3/1  "w4"
  Switch3/1 -> Sum/4, Bus Creator2/4
  incluir_din_motor/1 -> Switch/2, Switch1/2, Switch2/2, Switch3/2
  Mux/1 -> w1,w2,w3,w4/1
  U1d/1 -> Bus Creator1/1
  U2d/1 -> Bus Creator1/2
  U3d/1 -> Bus Creator1/3
  U4d/1 -> Bus Creator1/4

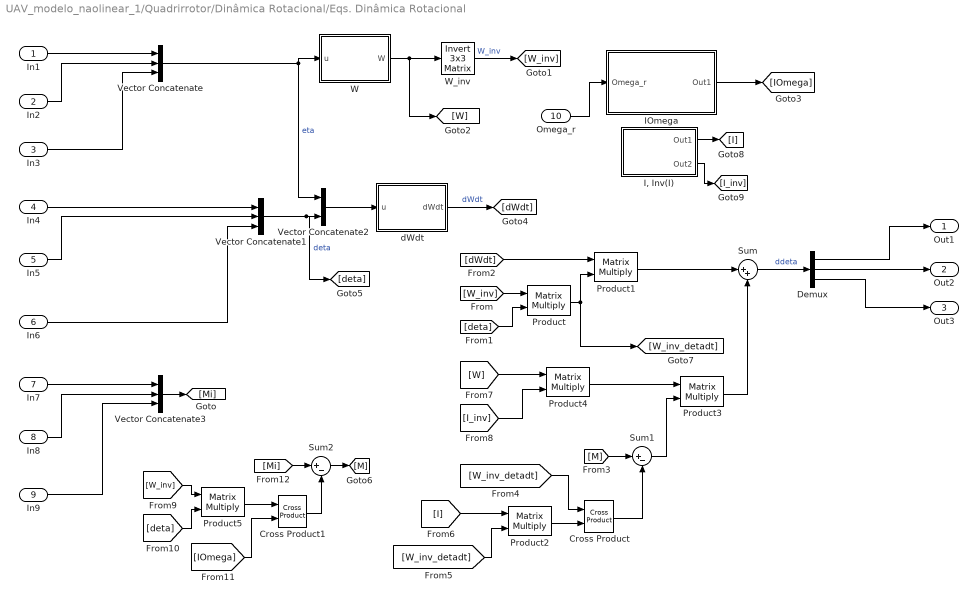
== system UAV_modelo_naolinear_1/Quadrirrotor/Dinâmica Rotacional/Eqs. Dinâmica Rotacional ==
  In1 : Inport
  In2 : Inport  Port=2
  In3 : Inport  Port=3
  In4 : Inport  Port=4
  In5 : Inport  Port=5
  In6 : Inport  Port=6
  In7 : Inport  Port=7
  In8 : Inport  Port=8
  In9 : Inport  Port=9
  Omega_r : Inport  Port=10
  Cross Product : vrlib/Utilities/Cross Product
      settings: SourceProductBaseCode=VR
  Cross Product1 : vrlib/Utilities/Cross Product
      settings: SourceProductBaseCode=VR
  Demux : Demux  Outputs=3
  "I, Inv(I)" : Subsystem
      mask Display:
      | port_label('output',1,'I')
      | port_label('output',2,'inv(I)')
  IOmega : Subsystem
      mask Display:
      | port_label('input',1,'Omega_r')
      | port_label('output',1,'IOmega')
  Product{,1..5} (6 alike) : Product  Multiplication=Matrix(*)
  Sum : Sum  Inputs=|++
  Sum1 : Sum  Inputs=|+-
  Sum2 : Sum  Inputs=|+-
  Vector Concatenate : Concatenate  NumInputs=3
  Vector Concatenate1 : Concatenate  NumInputs=3
  Vector Concatenate2 : Concatenate
  Vector Concatenate3 : Concatenate  NumInputs=3
  W : MATLAB Function  TreatAsAtomicUnit=on
  W_inv : aerolibutil/Invert  3x3 Matrix
  dWdt : MATLAB Function  TreatAsAtomicUnit=on
  Out1 : Outport
  Out2 : Outport  Port=2
  Out3 : Outport  Port=3
  wires:
  Vector Concatenate3/1 -> [Mi]
  W_inv/1 -> [W_inv]  "W_inv"
  [dWdt] -> Product1/1
  Vector Concatenate1/1 -> [deta], Vector Concatenate2/2  "deta"
  [Mi] -> Sum2/1
  Cross Product1/1 -> Sum2/2
  [W_inv] -> Product5/1
  [IOmega] -> Cross Product1/2
  Product5/1 -> Cross Product1/1
  [deta] -> Product5/2
  "I, Inv(I)"/1(Out1) -> [I]
  dWdt/1(dWdt) -> [dWdt]  "dWdt"
  In5/1 -> Vector Concatenate1/2
  In6/1 -> Vector Concatenate1/3
  In4/1 -> Vector Concatenate1/1
  In7/1 -> Vector Concatenate3/1
  In1/1 -> Vector Concatenate/1
  In2/1 -> Vector Concatenate/2
  In3/1 -> Vector Concatenate/3
  In8/1 -> Vector Concatenate3/2
  [deta] -> Product/2
  In9/1 -> Vector Concatenate3/3
  [W] -> Product4/1
  Sum2/1 -> [M]
  Product4/1 -> Product3/1
  Cross Product/1 -> Sum1/2
  [M] -> Sum1/1
  [I_inv] -> Product4/2
  [W_inv_detadt] -> Cross Product/1
  Product/1 -> [W_inv_detadt], Product1/2
  Product1/1 -> Sum/1
  [I] -> Product2/1
  [W_inv] -> Product/1
  [W_inv_detadt] -> Product2/2
  Sum/1 -> Demux/1  "ddeta"
  Demux/1 -> Out1/1
  Demux/2 -> Out2/1
  Product2/1 -> Cross Product/2
  Demux/3 -> Out3/1
  Product3/1 -> Sum/2
  IOmega/1(Out1) -> [IOmega]
  Vector Concatenate2/1 -> dWdt/1(u)
  Vector Concatenate/1 -> W/1(u), Vector Concatenate2/1  "eta"
  W/1(W) -> [W], W_inv/1
  Sum1/1 -> Product3/2
  "I, Inv(I)"/2(Out2) -> [I_inv]
  Omega_r/1 -> IOmega/1(Omega_r)

== system UAV_modelo_naolinear_1/Quadrirrotor/Motores do UAV /Motor DC 1 ==
  wd : Inport
  Modelo Motor 1 : TransferFcn  Numerator=[Kp]  Denominator=[tau_a 1]
  Transport Delay : TransportDelay  DelayTime=tau_s  PadeOrder=2
  w : Outport
  wires:
  Modelo Motor 1/1 -> Transport Delay/1
  Transport Delay/1 -> w/1  "w1"
  wd/1 -> Modelo Motor 1/1

== system UAV_modelo_naolinear_1/Quadrirrotor/Motores do UAV /Motor DC 2 ==
  In1 : Inport
  Modelo Motor 2 : TransferFcn  Numerator=[Kp]  Denominator=[tau_a 1]
  Transport Delay1 : TransportDelay  DelayTime=tau_s  PadeOrder=2
  Out1 : Outport
  wires:
  Modelo Motor 2/1 -> Transport Delay1/1
  In1/1 -> Modelo Motor 2/1
  Transport Delay1/1 -> Out1/1  "w2"

== system UAV_modelo_naolinear_1/Quadrirrotor/Motores do UAV /Motor DC 3 ==
  In1 : Inport
  Modelo Motor 3 : TransferFcn  Numerator=[Kp]  Denominator=[tau_a 1]
  Transport Delay2 : TransportDelay  DelayTime=tau_s  PadeOrder=2
  Out1 : Outport
  wires:
  In1/1 -> Modelo Motor 3/1
  Modelo Motor 3/1 -> Transport Delay2/1
  Transport Delay2/1 -> Out1/1  "w3"

== system UAV_modelo_naolinear_1/Quadrirrotor/Motores do UAV /Motor DC 4 ==
  In1 : Inport
  Modelo Motor 4 : TransferFcn  Numerator=[Kp]  Denominator=[tau_a 1]
  Transport Delay3 : TransportDelay  DelayTime=tau_s  PadeOrder=2
  Out1 : Outport
  wires:
  Modelo Motor 4/1 -> Transport Delay3/1
  In1/1 -> Modelo Motor 4/1
  Transport Delay3/1 -> Out1/1  "w4"

== system UAV_modelo_naolinear_1/Quadrirrotor/Dinâmica Rotacional/Eqs. Dinâmica Rotacional/I, Inv(I) ==
  Constant6 : Constant  Value=Ixx
  Constant7 : Constant  Value=Iyy
  Constant8 : Constant  Value=Izz
  Constant9 : Constant  Value=0
  I : sharedutil/Create 3x3 Matrix
  I_inv : aerolibutil/Invert  3x3 Matrix
  Out1 : Outport
  Out2 : Outport  Port=2
  wires:
  Constant9/1 -> I/2, I/3, I/4, I/6, I/7, I/8
  Constant8/1 -> I/9
  Constant7/1 -> I/5
  Constant6/1 -> I/1
  I_inv/1 -> Out2/1  "I_inv"
  I/1 -> Out1/1, I_inv/1  "I"

== system UAV_modelo_naolinear_1/Quadrirrotor/Dinâmica Rotacional/Eqs. Dinâmica Rotacional/IOmega ==
  Omega_r : Inport
  Constant10 : Constant  Value=Ir
  Constant12 : Constant  Value=0
  Product : Product
  Vector Concatenate3 : Concatenate  NumInputs=3
  Out1 : Outport
  wires:
  Constant10/1 -> Product/1
  Omega_r/1 -> Product/2
  Product/1 -> Vector Concatenate3/3
  Constant12/1 -> Vector Concatenate3/2, Vector Concatenate3/1
  Vector Concatenate3/1 -> Out1/1  "IOmega"

== matlab function UAV_modelo_naolinear_1/Quadrirrotor/Dinâmica Rotacional/Eqs. Dinâmica Rotacional/dWdt ==
  data: u input; dWdt output
function dWdt = fcn(u)
dWdt = zeros(3,3);
%#codegen
phi = u(1);
theta = u(2);
psi = u(3);
dphi = u(4);
dtheta = u(5);
dpsi = u(6);

dWdt(1,1) = 0;
dWdt(1,2) = (cos(phi)*cos(theta)*sin(theta)*dphi + sin(phi)*dtheta)/cos(theta)^2;
dWdt(1,3) = -(cos(theta)*sin(phi)*sin(theta)*dphi - cos(phi)*dtheta)/cos(theta)^2;
dWdt(2,1) = 0;
dWdt(2,2) = -sin(phi)*dphi;
dWdt(2,3) = -cos(phi)*dphi;
dWdt(3,1) = 0;
dWdt(3,2) = (cos(phi)*cos(theta)*dphi + sin(phi)*sin(theta)*dtheta)/cos(theta)^2;
dWdt(3,3) = -(cos(theta)*sin(phi)*dphi - cos(phi)*sin(theta)*dtheta)/cos(theta)^2;
%
%dWdt = [0,(cos(phi)*cos(theta)*sin(theta)*dphi + sin(phi)*dtheta)/cos(theta)^2,-(cos(theta)*sin(phi)*sin(theta)*dphi - cos(phi)*dtheta)/cos(theta)^2;
%    0, -sin(phi)*dphi, -cos(phi)*dphi;
%    0,(cos(phi)*cos(theta)*dphi + sin(phi)*sin(theta)*dtheta)/cos(theta)^2,-(cos(theta)*sin(phi)*dphi - cos(phi)*sin(theta)*dtheta)/cos(theta)^2];
end

== matlab function UAV_modelo_naolinear_1/Quadrirrotor/Dinâmica Rotacional/Eqs. Dinâmica Rotacional/W ==
  data: u input; W output
function W = fcn(u)
%#codegen
W = zeros(3,3);
phi = u(1);
theta = u(2);
psi = u(3);
W(1,1)= 1;
W(1,2)= sin(phi)*tan(theta);
W(1,3)= cos(phi)*tan(theta);
W(2,1)= 0;
W(2,2)= cos(phi);
W(2,3)= -sin(phi);
W(3,1)= 0;
W(3,2)= sin(phi)/cos(theta);
W(3,3)=  cos(phi)/cos(theta);
%
%W = [1, sin(phi)*tan(theta), cos(phi)*tan(theta);
%     0, cos(phi),  -sin(phi);
%     0, sin(phi)/cos(theta), cos(phi)/cos(theta)]; 
end
